simulink model "trab2_observador"  (R2023a)
settings: Solver=VariableStepAuto  StartTime=0.0  StopTime=10.0  RelTol=1e-3
values from neighbouring files (symbols this model uses):
  A = [[-3.333 0 -1.3333];[2 -2 0];[0 4.7727 -0.04545]]    [Controlador_t3.m]    (also in lab2_controle2.m = [[0 1 0];[981.0001 0 -2.8814];[0 0 -100]]; trab3_controle2.m; trabalho1_controle2.m = [[0 1];[0 0]])
  b = [0; 0; 100]    [lab2_controle2.m]    (also in trabalho1_controle2.m = [0;-0.294])
  c = [0 0 1]    [Controlador_t3.m]    (also in lab2_controle2.m = [1 0 0]; trab3_controle2.m; trabalho1_controle2.m = [1,0])
  kt2 = place(A,b,polos_desejados_2)    [lab2_controle2.m]
  Nbar = 1/ganhocc    [lab2_controle2.m]
  vetor_obs = place(A', c',polos_observador)    [lab2_controle2.m]
settings Model: Creator=wesle  LastModifiedBy=wesle

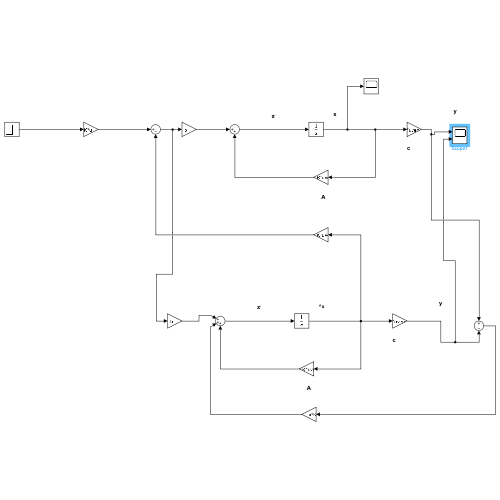
[thumbnail: Simulink's stored preview of the top-level diagram]
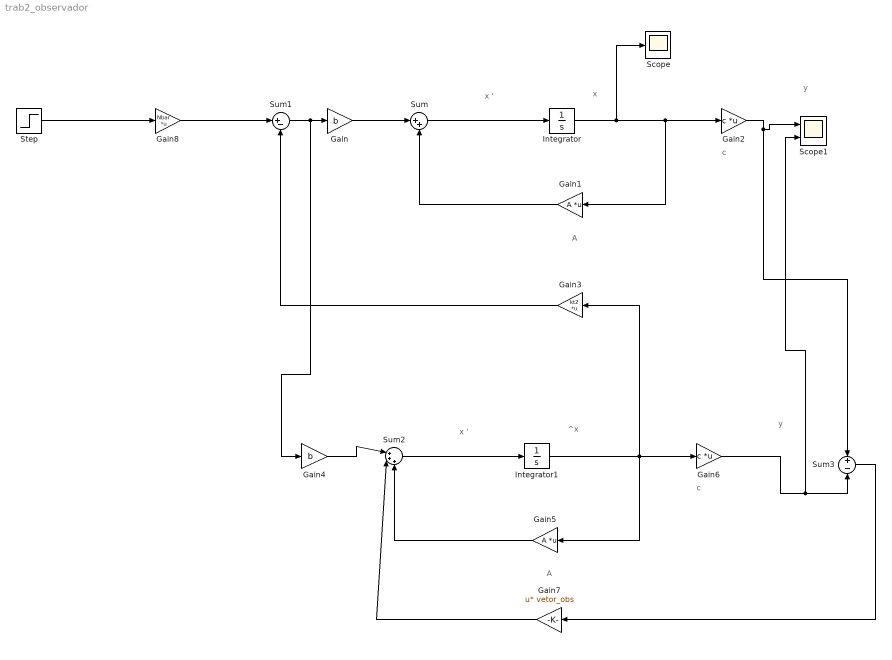
== system trab2_observador ==
  note: c
  note: A
  note: x '
  note: x
  note: y
  note: A
  note: y
  note: x '
  note: ^x
  note: c
  Gain : Gain  Gain=b
  Gain1 : Gain  Gain=A  Multiplication=Matrix(K*u) (u vector)
  Gain2 : Gain  Gain=c  Multiplication=Matrix(K*u) (u vector)
  Gain3 : Gain  Gain=kt2  Multiplication=Matrix(K*u) (u vector)
  Gain4 : Gain  Gain=b
  Gain5 : Gain  Gain=A  Multiplication=Matrix(K*u) (u vector)
  Gain6 : Gain  Gain=c  Multiplication=Matrix(K*u) (u vector)
  Gain7 : Gain  Gain=vetor_obs  Multiplication=Matrix(u*K)
  Gain8 : Gain  Gain=Nbar  Multiplication=Matrix(K*u)
  Integrator : Integrator  InitialCondition=[0.0005 0 0]
  Integrator1 : Integrator
  Scope : Scope
  Scope1 : Scope  NumInputPorts=2
  Step : Step  After=0  SampleTime=0
  Sum : Sum  Inputs=|++
  Sum1 : Sum  Inputs=|+-
  Sum2 : Sum  Inputs=|+++
  Sum3 : Sum  Inputs=+|-
  wires:
  Sum/1 -> Integrator/1
  Gain/1 -> Sum/1
  Gain1/1 -> Sum/2
  Integrator/1 -> Scope/1, Gain1/1, Gain2/1
  Gain2/1 -> Sum3/1, Scope1/1
  Gain3/1 -> Sum1/2
  Sum1/1 -> Gain4/1, Gain/1
  Gain4/1 -> Sum2/1
  Sum2/1 -> Integrator1/1
  Integrator1/1 -> Gain3/1, Gain5/1, Gain6/1
  Gain5/1 -> Sum2/3
  Gain7/1 -> Sum2/2
  Gain6/1 -> Scope1/2, Sum3/2
  Sum3/1 -> Gain7/1
  Step/1 -> Gain8/1
  Gain8/1 -> Sum1/1
